simulink model "pi_controller_model"  (R2023b)
settings: Solver=VariableStepAuto  StartTime=0.0  StopTime=30  RelTol=1e-3
settings Model: Creator=charl  LastModifiedBy=troyk

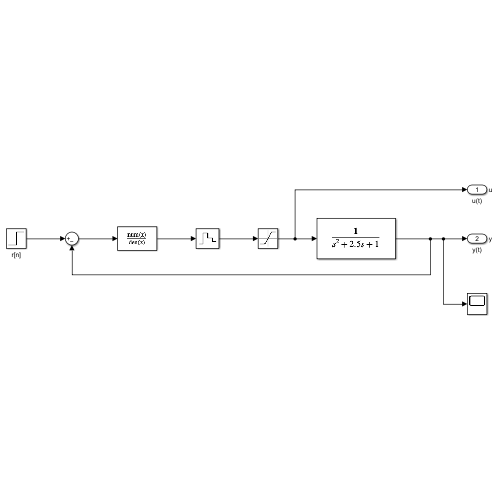
[thumbnail: Simulink's stored preview of the top-level diagram]
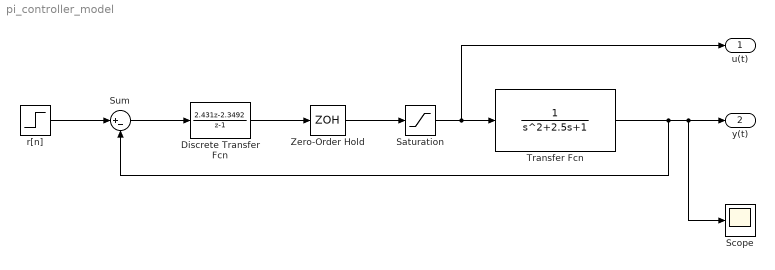
== system pi_controller_model ==
  Discrete Transfer Fcn : DiscreteTransferFcn  Numerator=[2.431 -2.3492]  Denominator=[1 -1]
  Saturation : Saturate  UpperLimit=5  LowerLimit=0
  Scope : Scope
  Sum : Sum  Inputs=|+-
  Transfer Fcn : TransferFcn  Denominator=[1 2.5 1]
  Zero-Order Hold : ZeroOrderHold  SampleTime=1/100
  r[n] : Step  Time=0  SampleTime=0
  u(t) : Outport  SignalName=u
  y(t) : Outport  Port=2  SignalName=y
  wires:
  Discrete Transfer Fcn/1 -> Zero-Order Hold/1
  Zero-Order Hold/1 -> Saturation/1
  r[n]/1 -> Sum/1
  Sum/1 -> Discrete Transfer Fcn/1
  Saturation/1 -> u(t)/1, Transfer Fcn/1
  Transfer Fcn/1 -> Sum/2, Scope/1, y(t)/1
